simulink model "Patient_PID_noDeadTime"  (R2022b)
settings: Solver=ode45  StartTime=0.0  StopTime=Tsim  FixedStep=Ts  RelTol=1e-15
values from neighbouring files (symbols this model uses):
  betaBIS = 2.13    [main_pfc.m]    (also in main_pfc_detail_analysis.m; main_pfc_pd_analysis.m; main_pid.m; main_pso.m)
  betaPSI = 2.13    [main_pfc.m]    (also in main_pfc_detail_analysis.m; main_pfc_pd_analysis.m; main_pid.m; main_pso.m)
  BIS_REF = 50    [main_pfc.m]    (also in main_pfc_detail_analysis.m; main_pfc_pd_analysis.m; main_pid.m; main_pso.m)
  C50N = 3.2425    [main_pfc.m]    (also in main_pfc_detail_analysis.m; main_pfc_pd_analysis.m; main_pid.m; main_pso.m)
  C50P = 4.16    [main_pfc.m]    (also in main_pfc_detail_analysis.m; main_pfc_pd_analysis.m; main_pid.m; main_pso.m)
  C50Pco = 8    [main_pfc.m]    (also in main_pfc_detail_analysis.m; main_pfc_pd_analysis.m; main_pid.m; main_pso.m)
  C50Pmap = 6    [main_pfc.m]    (also in main_pfc_detail_analysis.m; main_pfc_pd_analysis.m; main_pid.m; main_pso.m)
  C50R = 8.84    [main_pfc.m]    (also in main_pfc_detail_analysis.m; main_pfc_pd_analysis.m; main_pid.m; main_pso.m)
  C50Rco = 12    [main_pfc.m]    (also in main_pfc_detail_analysis.m; main_pfc_pd_analysis.m; main_pid.m; main_pso.m)
  C50Rmap = 17    [main_pfc.m]    (also in main_pfc_detail_analysis.m; main_pfc_pd_analysis.m; main_pid.m; main_pso.m)
  Cobasis = 5    [main_pfc.m]    (also in main_pfc_detail_analysis.m; main_pfc_pd_analysis.m; main_pid.m; main_pso.m)
  E0 = 100    [main_pfc.m]    (also in main_pfc_detail_analysis.m; main_pfc_pd_analysis.m; main_pid.m; main_pso.m)
  Emax = 100    [main_pfc.m]    (also in main_pfc_detail_analysis.m; main_pfc_pd_analysis.m; main_pid.m; main_pso.m)
  EmaxPco = 5    [main_pfc.m]    (also in main_pfc_detail_analysis.m; main_pfc_pd_analysis.m; main_pid.m; main_pso.m)
  EmaxPmap = 5    [main_pfc.m]    (also in main_pfc_detail_analysis.m; main_pfc_pd_analysis.m; main_pid.m; main_pso.m)
  EmaxRco = 5    [main_pfc.m]    (also in main_pfc_detail_analysis.m; main_pfc_pd_analysis.m; main_pid.m; main_pso.m)
  EmaxRmap = 70    [main_pfc.m]    (also in main_pfc_detail_analysis.m; main_pfc_pd_analysis.m; main_pid.m; main_pso.m)
  gainPco = 10    [main_pfc.m]    (also in main_pfc_detail_analysis.m; main_pfc_pd_analysis.m; main_pid.m; main_pso.m)
  gainPmap = 15    [main_pfc.m]    (also in main_pfc_detail_analysis.m; main_pfc_pd_analysis.m; main_pid.m; main_pso.m)
  gainRco = 10    [main_pfc.m]    (also in main_pfc_detail_analysis.m; main_pfc_pd_analysis.m; main_pid.m; main_pso.m)
  gainRmap = 10    [main_pfc.m]    (also in main_pfc_detail_analysis.m; main_pfc_pd_analysis.m; main_pid.m; main_pso.m)
  gamma = gammaBIS    (= 4)    [main_pfc.m]    (also in main_pfc_detail_analysis.m = exp_gamma(experiment); main_pfc_pd_analysis.m = exp_gamma(experiment); main_pid.m; main_pso.m)
  gammaBIS = 4    [main_pfc.m]    (also in main_pfc_detail_analysis.m; main_pfc_pd_analysis.m; main_pid.m; main_pso.m)
  gammaN = 2.6677    [main_pfc.m]    (also in main_pfc_detail_analysis.m; main_pfc_pd_analysis.m; main_pid.m; main_pso.m)
  gammaP = 2    [main_pfc.m]    (also in main_pfc_detail_analysis.m; main_pfc_pd_analysis.m; main_pid.m; main_pso.m)
  gammaPco = 4.5    [main_pfc.m]    (also in main_pfc_detail_analysis.m; main_pfc_pd_analysis.m; main_pid.m; main_pso.m)
  gammaPmap = 4.5    [main_pfc.m]    (also in main_pfc_detail_analysis.m; main_pfc_pd_analysis.m; main_pid.m; main_pso.m)
  gammaPSI = 4    [main_pfc.m]    (also in main_pfc_detail_analysis.m; main_pfc_pd_analysis.m; main_pid.m; main_pso.m)
  gammaR = 2.4    [main_pfc.m]    (also in main_pfc_detail_analysis.m; main_pfc_pd_analysis.m; main_pid.m; main_pso.m)
  gammaRco = 4.5    [main_pfc.m]    (also in main_pfc_detail_analysis.m; main_pfc_pd_analysis.m; main_pid.m; main_pso.m)
  gammaRmap = 4.5    [main_pfc.m]    (also in main_pfc_detail_analysis.m; main_pfc_pd_analysis.m; main_pid.m; main_pso.m)
  k0Pco = 0.81    [main_pfc.m]    (also in main_pfc_detail_analysis.m; main_pfc_pd_analysis.m; main_pid.m; main_pso.m)
  k0Pmap = 0.81    [main_pfc.m]    (also in main_pfc_detail_analysis.m; main_pfc_pd_analysis.m; main_pid.m; main_pso.m)
  k0r = 0.81    [main_pfc.m]    (also in main_pfc_detail_analysis.m; main_pfc_pd_analysis.m; main_pid.m; main_pso.m)
  k0Rco = 0.51    [main_pfc.m]    (also in main_pfc_detail_analysis.m; main_pfc_pd_analysis.m; main_pid.m; main_pso.m)
  k0Rmap = 0.31    [main_pfc.m]    (also in main_pfc_detail_analysis.m; main_pfc_pd_analysis.m; main_pid.m; main_pso.m)
  k1Pco = 0.81    [main_pfc.m]    (also in main_pfc_detail_analysis.m; main_pfc_pd_analysis.m; main_pid.m; main_pso.m)
  k1Pmap = 0.61    [main_pfc.m]    (also in main_pfc_detail_analysis.m; main_pfc_pd_analysis.m; main_pid.m; main_pso.m)
  k1r = 0.81    [main_pfc.m]    (also in main_pfc_detail_analysis.m; main_pfc_pd_analysis.m; main_pid.m; main_pso.m)
  k1Rco = 0.51    [main_pfc.m]    (also in main_pfc_detail_analysis.m; main_pfc_pd_analysis.m; main_pid.m; main_pso.m)
  k1Rmap = 0.31    [main_pfc.m]    (also in main_pfc_detail_analysis.m; main_pfc_pd_analysis.m; main_pid.m; main_pso.m)
  MAPbasis = 80    [main_pfc.m]    (also in main_pfc_detail_analysis.m; main_pfc_pd_analysis.m; main_pid.m; main_pso.m)
  sigma = sigmaBIS    (= 8.2)    [main_pfc.m]    (also in main_pfc_detail_analysis.m = exp_sigma(experiment); main_pfc_pd_analysis.m = exp_sigma(experiment); main_pid.m; main_pso.m)
  sigmaBIS = 8.2    [main_pfc.m]    (also in main_pfc_detail_analysis.m; main_pfc_pd_analysis.m; main_pid.m; main_pso.m)
  sigmaPSI = 8.2    [main_pfc.m]    (also in main_pfc_detail_analysis.m; main_pfc_pd_analysis.m; main_pid.m; main_pso.m)
  Ts = 1    [main_pfc.m]    (also in main_pfc_detail_analysis.m; main_pfc_pd_analysis.m; main_pid.m; main_pso.m)
undefined symbols (not defined in the file or in its folder): denRass, NOCI, numRass
libraries: cstblocks x11, slpidlib x1
settings Model: Creator=cionescu  LastModifiedBy=krist
settings SolverCC: AlgebraicLoopSolver=TrustRegion
settings DataIOCC: SaveState=on  ReturnWorkspaceOutputs=off
settings DebuggingCC: UnconnectedInputMsg=warning  UnconnectedOutputMsg=warning  UnconnectedLineMsg=warning  SFMachineParentedDataDiag=warning  ArithmeticOperatorsInVariantConditions=warning
settings ModelReferenceCC: EnableRefExpFcnMdlSchedulingChecks=on
settings SFSimCC: SimUseLocalCustomCode=off  CustomCodeUndefinedFunction=UseInterfaceOnly
settings RTWCC: RTWUseLocalCustomCode=off  DLArmComputeVersion=19.05
settings CodeAppCC: StateflowObjectComments=on

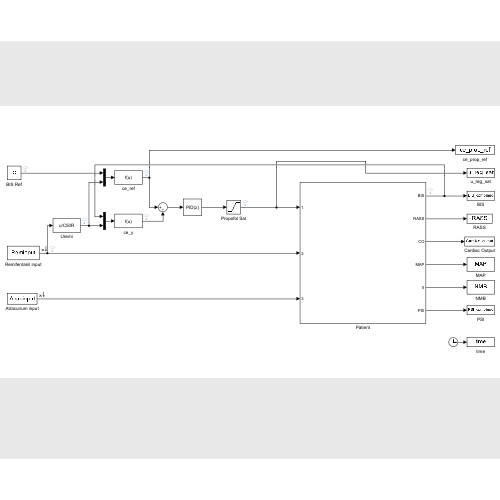
[thumbnail: Simulink's stored preview of the top-level diagram]
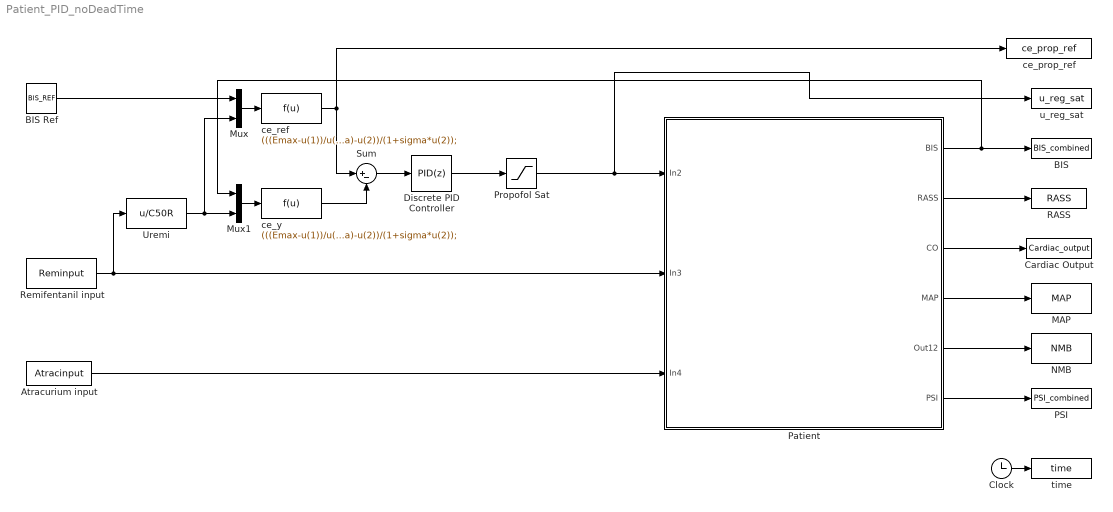
== system Patient_PID_noDeadTime ==
  Atracurium input : FromWorkspace  VariableName=Atracinput  Interpolate=off  OutputAfterFinalValue=Setting to zero
  BIS : ToWorkspace  VariableName=BIS_combined  SampleTime=1
      settings: Save2DSignal=2-D array (concatenate along first dimension)
  BIS Ref : Constant  Value=BIS_REF
  Cardiac Output : ToWorkspace  VariableName=Cardiac_output  SampleTime=1
      settings: Save2DSignal=2-D array (concatenate along first dimension)
  Clock : Clock
  Discrete PID Controller : slpidlib/PID Controller  Controller=PID  Form=Parallel  TimeDomain=Discrete-time  UseExternalTs=off  SampleTime=Ts  IntegratorMethod=Forward Euler  FilterMethod=Forward Euler  ControllerParametersSource=internal  P=3.22089409751815  I=0.565580688096251  UseKiTs=off  D=1.95772083863868  N=1.54022656452411  UseFilter=on  TunerSelectOption=Transfer Function Based (PID Tuner App)  InitialConditionSource=internal  InitialConditionForIntegrator=0  InitialConditionForFilter=0  DifferentiatorICPrevScaledInput=0  ExternalReset=none  TrackingMode=off  Kt=1  LimitOutput=off  SatLimitsSource=internal  UpperSaturationLimit=inf  LowerSaturationLimit=-inf  LinearizeAsGain=off  AntiWindupMode=none  Kb=1  LimitIntegrator=off  UpperIntegratorSaturationLimit=inf  LowerIntegratorSaturationLimit=-inf  POutMin=[]  POutMax=[]  IOutMin=[]  IOutMax=[]  DOutMin=[]  DOutMax=[]  NOutMin=[]  NOutMax=[]  SumOutMin=[]  SumOutMax=[]  SaturationOutMin=[]  SaturationOutMax=[]  PParamMin=[]  PParamMax=[]  IParamMin=[]  IParamMax=[]  DParamMin=[]  DParamMax=[]  NParamMin=[]  NParamMax=[]  KbParamMin=[]  KbParamMax=[]  KtParamMin=[]  KtParamMax=[]  KbOutMin=[]  KbOutMax=[]  KtOutMin=[]  KtOutMax=[]  IntegratorOutMin=[]  IntegratorOutMax=[]  FilterOutMin=[]  FilterOutMax=[]  SumI1OutMin=[]  SumI1OutMax=[]  SumI2OutMin=[]  SumI2OutMax=[]  SumI3OutMin=[]  SumI3OutMax=[]  SumI4OutMin=[]  SumI4OutMax=[]  SumDOutMin=[]  SumDOutMax=[]  DifferentiatorOutMin=[]  DifferentiatorOutMax=[]  FilterDiffOutCoefMin=[]  FilterDiffOutCoefMax=[]  ReciprocalOutMin=[]  ReciprocalOutMax=[]  SumDenOutMin=[]  SumDenOutMax=[]  SumNumOutMin=[]  SumNumOutMax=[]  DivideOutMin=[]  DivideOutMax=[]  UdiffTsProdOutMin=[]  UdiffTsProdOutMax=[]  NTsProdOutMin=[]  NTsProdOutMax=[]  UintegralTsProdOutMin=[]  UintegralTsProdOutMax=[]  UngainTsProdOutMin=[]  UngainTsProdOutMax=[]  ClampingZeroOutDataTypeStr=Inherit: Inherit via back propagation  ClampingZeroOutMin=[]  ClampingZeroOutMax=[]  FilterDenConstantOutDataTypeStr=Inherit: Inherit via back propagation  FilterDenConstantOutMin=[]  FilterDenConstantOutMax=[]  PCopyOutDataTypeStr=Inherit: Inherit via back propagation  PCopyOutMin=[]  PCopyOutMax=[]  NCopyOutDataTypeStr=Inherit: Inherit via back propagation  NCopyOutMin=[]  NCopyOutMax=[]  IntegratorContinuousStateAttributes=''  IntegratorStateMustResolveToSignalObject=off  IntegratorRTWStateStorageClass=Auto  FilterContinuousStateAttributes=''  FilterStateMustResolveToSignalObject=off  FilterRTWStateStorageClass=Auto  ParallelPVariant=InternalParameters  IdealPVariant=Disabled  IVariant=InternalParameters  DVariant=InternalParameters  IntegratorVariant=Discrete  SatVariant=Disabled  AWVariant=Passthrough  PCopyVariant=Disabled  TRVariant=Disabled  FdbkBlocksVariant=Forward  IdealPFdbkVariant=Disabled  SatFdbkVariant=Disabled  DerivativeFilterVariant=ForwardEulerFilter  NVariant=InternalParameters  NCopyVariant=Disabled  FilterICVariant=InternalICsFilter  IntegratorICVariant=InternalICs  ExternalResetVariant=Disabled  TRSumVariant=Passthrough  SumFdbkVariant=Disabled  SumVariant=Sum_PID  TsampFilterVariant=InternalTs  TsampNgainVariant=Passthrough  TsampIntegralVariant=Passthrough  ExternalSaturationOutDataTypeStr=Inherit: Same as second input
      settings: LibrarySourceBlock=simulink/Discrete/Discrete PID Controller
  MAP : ToWorkspace  VariableName=MAP  SampleTime=1
      settings: Save2DSignal=2-D array (concatenate along first dimension)
  Mux : Mux  Inputs=2
  Mux1 : Mux  Inputs=2
  NMB : ToWorkspace  VariableName=NMB  SampleTime=1
      settings: Save2DSignal=2-D array (concatenate along first dimension)
  PSI : ToWorkspace  VariableName=PSI_combined  SampleTime=1
      settings: Save2DSignal=2-D array (concatenate along first dimension)
  Patient : Subsystem
  Propofol Sat : Saturate  UpperLimit=6  LowerLimit=0
  RASS : ToWorkspace  VariableName=RASS  SampleTime=1
      settings: Save2DSignal=2-D array (concatenate along first dimension)
  Remifentanil input : FromWorkspace  VariableName=Reminput  Interpolate=off  OutputAfterFinalValue=Setting to zero
  Sum : Sum  Inputs=|+-
  Uremi : Fcn  Expr=u/C50R
  ce_prop_ref : ToWorkspace  VariableName=ce_prop_ref  SampleTime=1
      settings: Save2DSignal=2-D array (concatenate along first dimension)
  ce_ref : Fcn  Expr=(((Emax-u(1))/u(1))^(1/gamma)-u(2))/(1+sigma*u(2));
  ce_y : Fcn  Expr=(((Emax-u(1))/u(1))^(1/gamma)-u(2))/(1+sigma*u(2));
  time : ToWorkspace  VariableName=time  SampleTime=1
      settings: Save2DSignal=2-D array (concatenate along first dimension)
  u_reg_sat : ToWorkspace  VariableName=u_reg_sat  SampleTime=1
      settings: Save2DSignal=2-D array (concatenate along first dimension)
  wires:
  Remifentanil input/1 -> Patient/2(In3), Uremi/1
  Atracurium input/1 -> Patient/3(In4)
  Patient/2(RASS) -> RASS/1
  Patient/3(CO) -> Cardiac Output/1
  Patient/4(MAP) -> MAP/1
  Patient/5(Out12) -> NMB/1
  Patient/6(PSI) -> PSI/1
  Clock/1 -> time/1
  Patient/1(BIS) -> Mux1/1, BIS/1
  Mux/1 -> ce_ref/1
  Uremi/1 -> Mux/2, Mux1/2
  BIS Ref/1 -> Mux/1
  Mux1/1 -> ce_y/1
  Discrete PID Controller/1 -> Propofol Sat/1
  ce_ref/1 -> Sum/1, ce_prop_ref/1
  Sum/1 -> Discrete PID Controller/1
  Propofol Sat/1 -> u_reg_sat/1, Patient/1(In2)
  ce_y/1 -> Sum/2

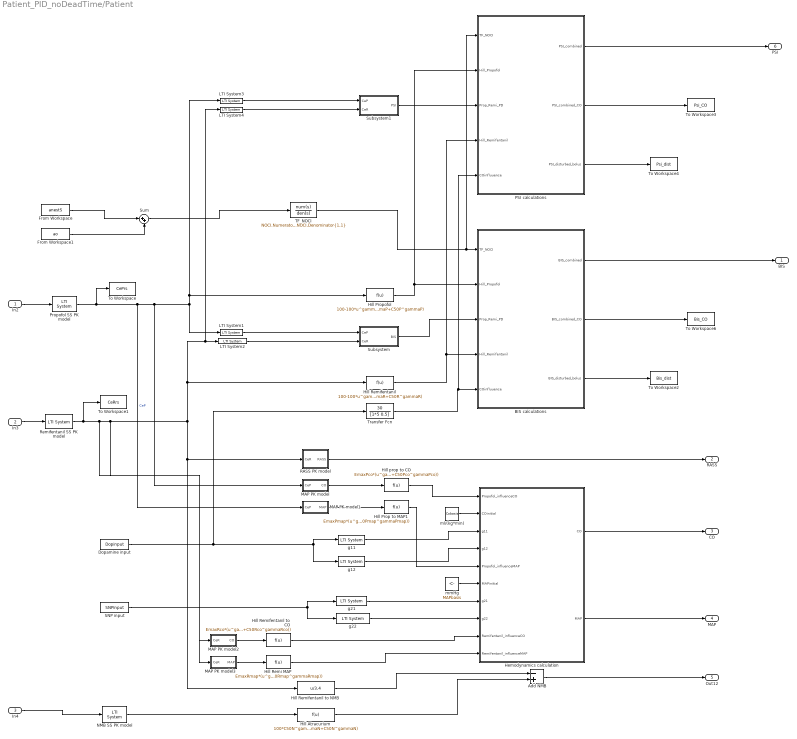
== system Patient_PID_noDeadTime/Patient ==
  In2 : Inport
  In3 : Inport  Port=2
  In4 : Inport  Port=3
  Add NMB : Sum  Inputs=-+
  BIS calculations : MATLAB Function  TreatAsAtomicUnit=on
  Dopamine input : FromWorkspace  VariableName=Dopinput  Interpolate=off  OutputAfterFinalValue=Setting to zero
  From Workspace : FromWorkspace  VariableName=anestS
  From Workspace1 : FromWorkspace  VariableName=ao
  Hemodynamics calculation : MATLAB Function  TreatAsAtomicUnit=on
  Hill Atracurium : Fcn  Expr=100*C50N^gammaN/(u^gammaN+C50N^gammaN)
  Hill Prop to MAP1 : Fcn  Expr=EmaxPmap*(u^gammaPmap/(u^gammaPmap+C50Pmap^gammaPmap))
  Hill Propofol : Fcn  Expr=100-100*u^gammaP/(u^gammaP+C50P^gammaP)
  Hill Remi MAP : Fcn  Expr=EmaxRmap*(u^gammaRmap/(u^gammaRmap+C50Rmap^gammaRmap))
  Hill Remifentanil : Fcn  Expr=100-100*u^gammaR/(u^gammaR+C50R^gammaR)
  Hill Remifentanil to CO : Fcn  Expr=EmaxRco*(u^gammaRco/(u^gammaRco+C50Rco^gammaRco))
  Hill Remifentanil to NMB : Fcn  Expr=u/3.4
  Hill prop to CO : Fcn  Expr=EmaxPco*(u^gammaPco/(u^gammaPco+C50Pco^gammaPco))
  LTI System1 : cstblocks/LTI System  sys=dBIS  IC=[]
  LTI System2 : cstblocks/LTI System  sys=dBIS  IC=[]
  LTI System3 : cstblocks/LTI System  sys=dPSI  IC=[]
  LTI System4 : cstblocks/LTI System  sys=dPSI  IC=[]
  MAP PK model : Subsystem
  MAP PK model1 : Subsystem
  MAP PK model2 : Subsystem
  MAP PK model3 : Subsystem
  NMB SS PK model : cstblocks/LTI System  sys=nmbSS  IC=[0;0;0]
  PSI calculations : MATLAB Function  TreatAsAtomicUnit=on
  Propofol SS PK model : cstblocks/LTI System  sys=propSS  IC=0
  RASS PK model : Subsystem
  Remifentanil SS PK model : cstblocks/LTI System  sys=remiSS  IC=0
  SNP input : FromWorkspace  VariableName=SNPinput  Interpolate=off  OutputAfterFinalValue=Setting to zero
  Subsystem : Subsystem
  Subsystem1 : Subsystem
  Sum : Sum  Inputs=|++
  TF_NOCI : TransferFcn  Numerator=NOCI.Numerator{1,1}  Denominator=NOCI.Denominator{1,1}
  To Workspace : ToWorkspace  VariableName=CePrs  SampleTime=1
      settings: Save2DSignal=2-D array (concatenate along first dimension)
  To Workspace1 : ToWorkspace  VariableName=CeRrs  SampleTime=-1
      settings: Save2DSignal=2-D array (concatenate along first dimension)
  To Workspace2 : ToWorkspace  VariableName=Bis_dist  SampleTime=1
      settings: Save2DSignal=2-D array (concatenate along first dimension)
  To Workspace3 : ToWorkspace  VariableName=Psi_CO  SampleTime=1
      settings: Save2DSignal=2-D array (concatenate along first dimension)
  To Workspace4 : ToWorkspace  VariableName=Psi_dist  SampleTime=1
      settings: Save2DSignal=2-D array (concatenate along first dimension)
  To Workspace6 : ToWorkspace  VariableName=Bis_CO  SampleTime=1
      settings: Save2DSignal=2-D array (concatenate along first dimension)
  Transfer Fcn : TransferFcn  Numerator=[30]  Denominator=[1*5 0.5]
  g11 : cstblocks/LTI System  sys=g11  IC=[]
  g12 : cstblocks/LTI System  sys=g12  IC=[]
  g21 : cstblocks/LTI System  sys=g21  IC=[]
  g22 : cstblocks/LTI System  sys=g22  IC=[]
  ml/(kg*min) : Constant  Value=Cobasis  SampleTime=Ts
  mmHg : Constant  Value=MAPbasis  SampleTime=Ts
  BIS : Outport
  RASS : Outport  Port=2
  CO : Outport  Port=3
  MAP : Outport  Port=4
  Out12 : Outport  Port=5
  PSI : Outport  Port=6
  wires:
  Remifentanil SS PK model/1 -> To Workspace1/1, MAP PK model2/1(CeR), MAP PK model3/1(CeR), Hill Remifentanil to NMB/1, RASS PK model/1(CeR), LTI System4/1, LTI System2/1, Hill Remifentanil/1
  Dopamine input/1 -> Transfer Fcn/1, g12/1, g11/1
  Hill Remifentanil/1 -> PSI calculations/4(Hill_Remifentanil), BIS calculations/4(Hill_Remifentanil)
  LTI System2/1 -> Subsystem/2(CeR)
  Hill Remifentanil to NMB/1 -> Add NMB/1
  Hill prop to CO/1 -> Hemodynamics calculation/1(Propofol_influenceCO)
  Hill Prop to MAP1/1 -> Hemodynamics calculation/5(Propofol_influenceMAP)
  Propofol SS PK model/1 -> To Workspace/1, MAP PK model1/1(CeP), MAP PK model/1(CeP), LTI System3/1, Hill Propofol/1, LTI System1/1  "CeP"
  g12/1 -> Hemodynamics calculation/4(g12)
  Hill Atracurium/1 -> Add NMB/2
  MAP PK model/1(CO) -> Hill prop to CO/1
  SNP input/1 -> g22/1, g21/1
  In4/1 -> NMB SS PK model/1
  mmHg/1 -> Hemodynamics calculation/6(MAPinitial)
  g22/1 -> Hemodynamics calculation/8(g22)
  NMB SS PK model/1 -> Hill Atracurium/1
  Hill Propofol/1 -> BIS calculations/2(Hill_Propofol), PSI calculations/2(Hill_Propofol)
  In2/1 -> Propofol SS PK model/1
  Subsystem/1(BIS) -> BIS calculations/3(Prop_Remi_PD)
  Add NMB/1 -> Out12/1
  ml/(kg*min)/1 -> Hemodynamics calculation/2(COinitial)
  g21/1 -> Hemodynamics calculation/7(g21)
  LTI System1/1 -> Subsystem/1(CeP)
  g11/1 -> Hemodynamics calculation/3(g11)
  Hemodynamics calculation/1(CO) -> CO/1
  MAP PK model1/1(MAP) -> Hill Prop to MAP1/1
  Hemodynamics calculation/2(MAP) -> MAP/1
  In3/1 -> Remifentanil SS PK model/1
  RASS PK model/1(RASS) -> RASS/1
  MAP PK model2/1(CO) -> Hill Remifentanil to CO/1
  Hill Remifentanil to CO/1 -> Hemodynamics calculation/9(Remifentanil_influenceCO)
  Hill Remi MAP/1 -> Hemodynamics calculation/10(Remifentanil_influenceMAP)
  MAP PK model3/1(MAP) -> Hill Remi MAP/1
  Transfer Fcn/1 -> PSI calculations/5(COinfluuence), BIS calculations/5(COinfluuence)
  BIS calculations/2(BIS_combined_CO) -> To Workspace6/1
  BIS calculations/1(BIS_combined) -> BIS/1
  BIS calculations/3(BIS_disturbed_bolus) -> To Workspace2/1
  From Workspace/1 -> Sum/1
  From Workspace1/1 -> Sum/2
  Sum/1 -> TF_NOCI/1
  Subsystem1/1(PSI) -> PSI calculations/3(Prop_Remi_PD)
  TF_NOCI/1 -> PSI calculations/1(TF_NOCI), BIS calculations/1(TF_NOCI)
  PSI calculations/1(PSI_combined) -> PSI/1
  PSI calculations/2(PSI_combined_CO) -> To Workspace3/1
  PSI calculations/3(PSI_disturbed_bolus) -> To Workspace4/1
  LTI System3/1 -> Subsystem1/1(CeP)
  LTI System4/1 -> Subsystem1/2(CeR)

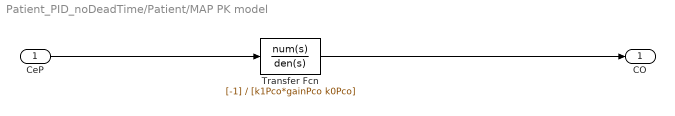
== system Patient_PID_noDeadTime/Patient/MAP PK model ==
  CeP : Inport
  Transfer Fcn : TransferFcn  Numerator=[-1]  Denominator=[k1Pco*gainPco k0Pco]
  CO : Outport
  wires:
  Transfer Fcn/1 -> CO/1
  CeP/1 -> Transfer Fcn/1

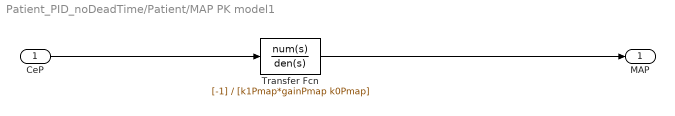
== system Patient_PID_noDeadTime/Patient/MAP PK model1 ==
  CeP : Inport
  Transfer Fcn : TransferFcn  Numerator=[-1]  Denominator=[k1Pmap*gainPmap k0Pmap]
  MAP : Outport
  wires:
  Transfer Fcn/1 -> MAP/1
  CeP/1 -> Transfer Fcn/1

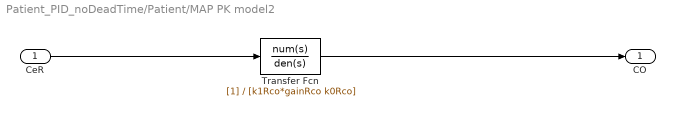
== system Patient_PID_noDeadTime/Patient/MAP PK model2 ==
  CeR : Inport
  Transfer Fcn : TransferFcn  Denominator=[k1Rco*gainRco k0Rco]
  CO : Outport
  wires:
  Transfer Fcn/1 -> CO/1
  CeR/1 -> Transfer Fcn/1

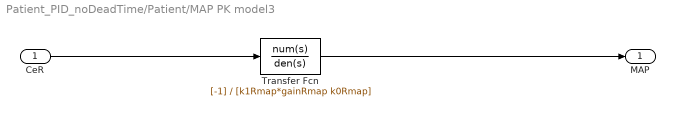
== system Patient_PID_noDeadTime/Patient/MAP PK model3 ==
  CeR : Inport
  Transfer Fcn : TransferFcn  Numerator=[-1]  Denominator=[k1Rmap*gainRmap k0Rmap]
  MAP : Outport
  wires:
  Transfer Fcn/1 -> MAP/1
  CeR/1 -> Transfer Fcn/1

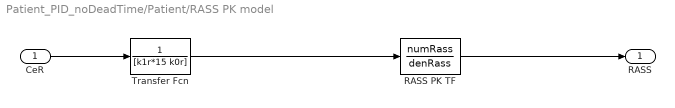
== system Patient_PID_noDeadTime/Patient/RASS PK model ==
  CeR : Inport
  RASS PK TF : TransferFcn  Numerator=numRass  Denominator=denRass
  Transfer Fcn : TransferFcn  Denominator=[k1r*15 k0r]
  RASS : Outport
  wires:
  CeR/1 -> Transfer Fcn/1
  Transfer Fcn/1 -> RASS PK TF/1
  RASS PK TF/1 -> RASS/1

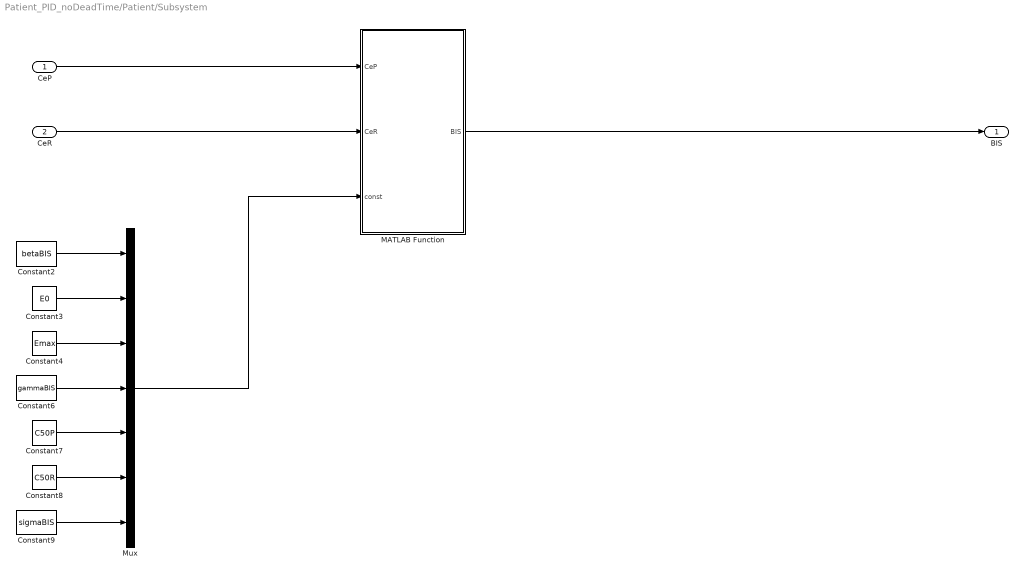
== system Patient_PID_noDeadTime/Patient/Subsystem ==
  CeP : Inport
  CeR : Inport  Port=2
  Constant2 : Constant  Value=betaBIS
  Constant3 : Constant  Value=E0
  Constant4 : Constant  Value=Emax
  Constant6 : Constant  Value=gammaBIS
  Constant7 : Constant  Value=C50P
  Constant8 : Constant  Value=C50R
  Constant9 : Constant  Value=sigmaBIS
  MATLAB Function : MATLAB Function  TreatAsAtomicUnit=on
  Mux : Mux  Inputs=7
  BIS : Outport
  wires:
  Constant9/1 -> Mux/7
  Constant8/1 -> Mux/6
  Constant4/1 -> Mux/3
  Mux/1 -> MATLAB Function/3(const)
  Constant7/1 -> Mux/5
  Constant3/1 -> Mux/2
  Constant6/1 -> Mux/4
  Constant2/1 -> Mux/1
  MATLAB Function/1(BIS) -> BIS/1
  CeP/1 -> MATLAB Function/1(CeP)
  CeR/1 -> MATLAB Function/2(CeR)

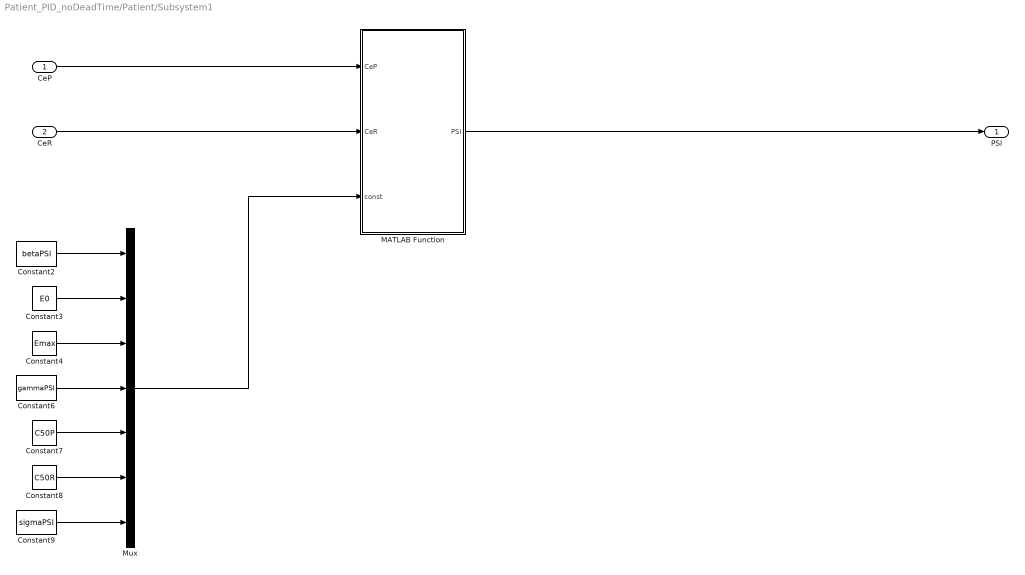
== system Patient_PID_noDeadTime/Patient/Subsystem1 ==
  CeP : Inport
  CeR : Inport  Port=2
  Constant2 : Constant  Value=betaPSI  VectorParams1D=off
  Constant3 : Constant  Value=E0
  Constant4 : Constant  Value=Emax
  Constant6 : Constant  Value=gammaPSI
  Constant7 : Constant  Value=C50P
  Constant8 : Constant  Value=C50R
  Constant9 : Constant  Value=sigmaPSI
  MATLAB Function : MATLAB Function  TreatAsAtomicUnit=on
  Mux : Mux  Inputs=7
  PSI : Outport
  wires:
  CeR/1 -> MATLAB Function/2(CeR)
  CeP/1 -> MATLAB Function/1(CeP)
  MATLAB Function/1(PSI) -> PSI/1
  Constant2/1 -> Mux/1
  Constant6/1 -> Mux/4
  Constant3/1 -> Mux/2
  Constant7/1 -> Mux/5
  Mux/1 -> MATLAB Function/3(const)
  Constant4/1 -> Mux/3
  Constant8/1 -> Mux/6
  Constant9/1 -> Mux/7

== matlab function Patient_PID_noDeadTime/Patient/Hemodynamics calculation ==
  data: Propofol_influenceCO input; COinitial input; g11 input; g12 input; Propofol_influenceMAP input; CO output; MAPinitial input; g21 input; MAP output; g22 input; Remifentanil_influenceCO input; Remifentanil_influenceMAP input
function [CO, MAP] = calculateHemodynamics(Propofol_influenceCO, COinitial, g11, g12, Propofol_influenceMAP, MAPinitial, g21, g22,Remifentanil_influenceCO,Remifentanil_influenceMAP)
CO = COinitial + g11 + g21+Propofol_influenceCO+Remifentanil_influenceCO;
MAP = MAPinitial + g12 + g22 +Propofol_influenceMAP+Remifentanil_influenceMAP;

== matlab function Patient_PID_noDeadTime/Patient/Subsystem/MATLAB Function ==
  data: CeP input; BIS output; CeR input; const input
function BIS = fcn(CeP,CeR, const)

if CeP >=0 && CeR >=0
%% Constant declaration
beta = const(1);
E0 = const(2)-100;
Emax = const(3);
gamma = const(4);
C50P = const(5);
C50R = const(6);
sigma = const(7);

%% 2D Calculations
Uprop=CeP./C50P; Uremi=CeR./C50R;
BIS=Emax - Emax*((Uprop)+(Uremi)+sigma*(Uprop)*(Uremi))^(gamma)/(1+(Uprop+Uremi+sigma*Uprop*Uremi)^(gamma));

else
    BIS = 100;
end

== matlab function Patient_PID_noDeadTime/Patient/BIS calculations ==
  data: TF_NOCI input; BIS_combined output; Hill_Propofol input; Prop_Remi_PD input; Hill_Remifentanil input; COinfluuence input; BIS_combined_CO output; BIS_disturbed_bolus output
% function [BIS_disturbed_single, BIS_output, BIS_disturbed, BIS_all, BIS_combined, BIS_combined_disturbed,BIS_combined_CO] = calculateBIS(TF_NOCI, Hill_Propofol, Prop_Remi_PD, Hill_Remifentanil,COinfluuence)
% % BIS_disturbed_single = TF_NOCI + Hill_Propofol;
% % BIS_output = Hill_Propofol;
% % BIS_disturbed = TF_NOCI + Prop_Remi_PD;
% % BIS_all = [Hill_Propofol,Prop_Remi_PD,Hill_Remifentanil];
% BIS_combined = Prop_Remi_PD;
% BIS_combined_CO= Prop_Remi_PD+COinfluuence;
% % BIS_combined_disturbed = TF_NOCI + Prop_Remi_PD;


function [BIS_combined, BIS_combined_CO,BIS_disturbed_bolus] = calculateBIS(TF_NOCI,Hill_Propofol, Prop_Remi_PD, Hill_Remifentanil,COinfluuence)
BIS_combined = Prop_Remi_PD;
BIS_disturbed_bolus = TF_NOCI + Prop_Remi_PD;
BIS_combined_CO= Prop_Remi_PD+COinfluuence;

== matlab function Patient_PID_noDeadTime/Patient/Subsystem1/MATLAB Function ==
  data: CeP input; PSI output; CeR input; const input
function PSI = fcn(CeP,CeR, const)

if CeP >=0 && CeR >=0
%% Constant declaration
beta = const(1);
E0 = const(2)-100;
Emax = const(3);
gamma = const(4);
C50P = const(5);
C50R = const(6);
sigma = const(7);

%% 2D Calculations
Uprop=CeP./C50P; Uremi=CeR./C50R;
PSI=Emax - Emax*((Uprop)+(Uremi)+sigma*(Uprop)*(Uremi))^(gamma)/(1+(Uprop+Uremi+sigma*Uprop*Uremi)^(gamma));

else
    PSI = 100;
end

== matlab function Patient_PID_noDeadTime/Patient/PSI calculations ==
  data: TF_NOCI input; PSI_combined output; Hill_Propofol input; Prop_Remi_PD input; Hill_Remifentanil input; COinfluuence input; PSI_combined_CO output; PSI_disturbed_bolus output
% function [PSI_disturbed_single, PSI_output, PSI_disturbed, PSI_all, PSI_combined, PSI_combined_disturbed,PSI_combined_CO] = calculatePSI(TF_NOCI, Hill_Propofol, Prop_Remi_PD, Hill_Remifentanil,COinfluuence)
% % PSI_disturbed_single = TF_NOCI + Hill_Propofol;
% % PSI_output = Hill_Propofol;
% % PSI_disturbed = TF_NOCI + Prop_Remi_PD;
% % PSI_all = [Hill_Propofol,Prop_Remi_PD,Hill_Remifentanil];
% PSI_combined = Prop_Remi_PD;
% PSI_combined_CO= Prop_Remi_PD+COinfluuence;
% % PSI_combined_disturbed = TF_NOCI + Prop_Remi_PD;


function [PSI_combined, PSI_combined_CO,PSI_disturbed_bolus] = calculatePSI(TF_NOCI,Hill_Propofol, Prop_Remi_PD, Hill_Remifentanil,COinfluuence)
PSI_combined = Prop_Remi_PD;
PSI_disturbed_bolus = TF_NOCI + Prop_Remi_PD;
PSI_combined_CO= Prop_Remi_PD+COinfluuence;
